simulink library "SEMACE4_OUT"  (R2021b)
settings: Solver=VariableStepAuto  StartTime=0.0  StopTime=10.0  RelTol=1e-3
settings Model: Creator=ACH  LastModifiedBy=ACH

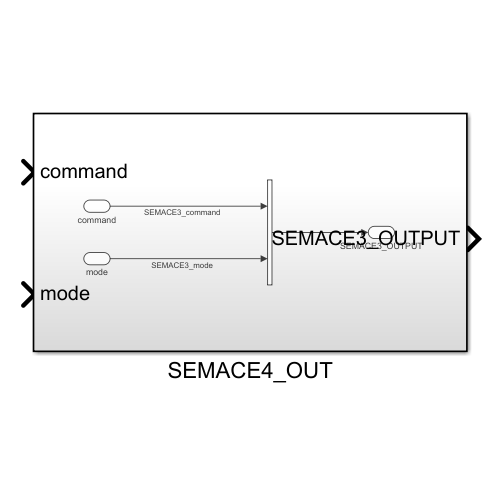
[thumbnail: Simulink's stored preview of the top-level diagram]
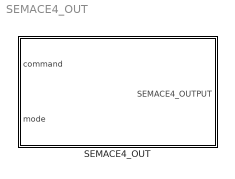
== system SEMACE4_OUT ==
  SEMACE4_OUT : Subsystem

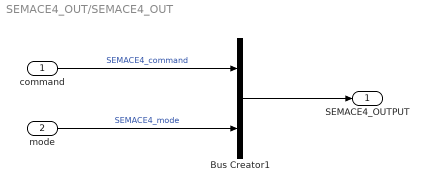
== system SEMACE4_OUT/SEMACE4_OUT ==
  command : Inport
  mode : Inport  Port=2
  Bus Creator1 : BusCreator  Inputs=2  OutDataTypeStr=Bus: SEMACE4_OUTPUT
  SEMACE4_OUTPUT : Outport  OutDataTypeStr=Bus: SEMACE4_OUTPUT
  wires:
  command/1 -> Bus Creator1/1  "SEMACE4_command"
  mode/1 -> Bus Creator1/2  "SEMACE4_mode"
  Bus Creator1/1 -> SEMACE4_OUTPUT/1
